simulink model "PIL_Block"  (R2017a)
settings: Solver=FixedStepAuto  StartTime=0.0  StopTime=50  FixedStep=0.01  RelTol=1e-3  EnableMultiTasking=on
libraries: pil_lib x1
settings Model: Creator=Administrator  LastModifiedBy=Administrator
settings OptimizationCC: PassReuseOutputArgsAs=Individual arguments  MaxStackSize=64
settings DebuggingCC: ParameterTunabilityLossMsg=error
settings HardwareCC: ProdBitPerPointer=32  ProdBitPerSizeT=32  ProdBitPerPtrDiffT=32  ProdLargestAtomicInteger=Long  ProdLargestAtomicFloat=Double  ProdWordSize=32  ProdHWDeviceType=ARM Compatible->ARM Cortex
settings SFSimCC: MATLABDynamicMemAlloc=off
settings RTWCC: SystemTargetFile=ert.tlc  HardwareBoard=ARM Cortex-M3 (QEMU)  TLCOptions=-aInlineSetEventsForThisBaseRateFcn=TLC_FALSE -aSuppressMultiTaskScheduler=TLC_FALSE -aRateBasedStepFcn=1  TemplateMakefile=ert_default_tmf  Description=Embedded Coder  GenerateReport=on  Toolchain=GNU Tools for ARM Embedded Processors  IncludeHyperlinkInReport=on  LaunchReport=on  CreateSILPILBlock=PIL  GenerateTraceInfo=on  GenerateTraceReport=on  GenerateTraceReportSl=on  GenerateTraceReportSf=on  GenerateTraceReportEml=on
settings CodeAppCC: ForceParamTrailComments=on  IgnoreCustomStorageClasses=off  OperatorAnnotations=on  SimulinkDataObjDesc=on  SFDataObjDesc=on  MATLABFcnDesc=on  InsertBlockDesc=on  MATLABSourceComments=on

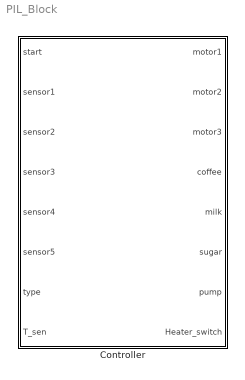
== system PIL_Block ==
  Controller : Subsystem  DialogController=pil_create_dialog  LoadFcn=|
      | try
      |    if ~strcmp(rtw.pil.getPILVersion, '6.12 (R2017a)_12')
      |       set_param(gcb, 'DialogController', '');
      |       set_param(gcb, 'DialogControllerArgs', '');
      |    end
      | catch e
      |       set_param(gcb, 'DialogController', '');
      |       set_param(gcb, 'DialogControllerArgs', '');
      | end
      mask help: PIL:pil:XILBlockMaskDesc
      mask Display: disp('PIL');

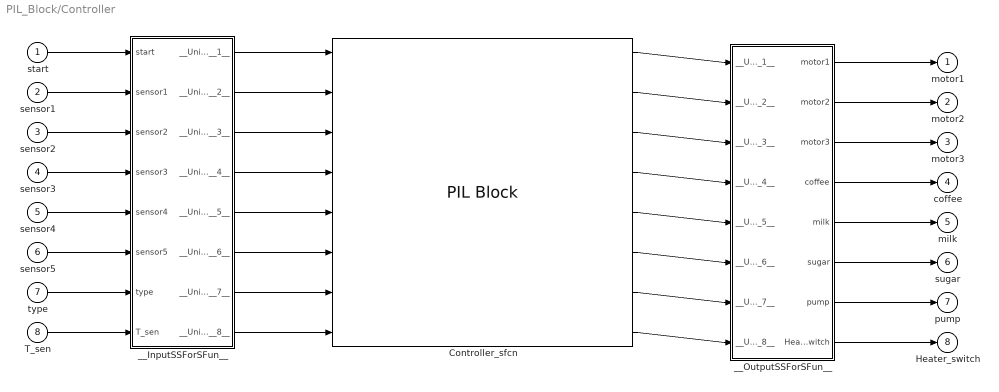
== system PIL_Block/Controller ==
  start : Inport
  sensor1 : Inport  Port=2
  sensor2 : Inport  Port=3
  sensor3 : Inport  Port=4
  sensor4 : Inport  Port=5
  sensor5 : Inport  Port=6
  type : Inport  Port=7
  T_sen : Inport  Port=8
  Controller_sfcn : pil_lib/PIL Block  SimulationMode=PIL  IsTopModelPIL=off  CodeDir=C:\Users\Administrator\Documents\MATLAB\Controller_ert_rtw  ConfigName=ARM Cortex-M3 (QEMU)  XrelIsTopModelCode=on
  __InputSSForSFun__ : Subsystem
  __OutputSSForSFun__ : Subsystem
  motor1 : Outport
  motor2 : Outport  Port=2
  motor3 : Outport  Port=3
  coffee : Outport  Port=4
  milk : Outport  Port=5
  sugar : Outport  Port=6
  pump : Outport  Port=7
  Heater_switch : Outport  Port=8
  wires:
  start/1 -> __InputSSForSFun__/1(start)
  sensor1/1 -> __InputSSForSFun__/2(sensor1)
  sensor2/1 -> __InputSSForSFun__/3(sensor2)
  sensor3/1 -> __InputSSForSFun__/4(sensor3)
  sensor4/1 -> __InputSSForSFun__/5(sensor4)
  sensor5/1 -> __InputSSForSFun__/6(sensor5)
  type/1 -> __InputSSForSFun__/7(type)
  T_sen/1 -> __InputSSForSFun__/8(T_sen)
  __InputSSForSFun__/1(__UniqueOutportName__1__) -> Controller_sfcn/1
  __InputSSForSFun__/2(__UniqueOutportName__2__) -> Controller_sfcn/2
  __InputSSForSFun__/3(__UniqueOutportName__3__) -> Controller_sfcn/3
  __InputSSForSFun__/4(__UniqueOutportName__4__) -> Controller_sfcn/4
  __InputSSForSFun__/5(__UniqueOutportName__5__) -> Controller_sfcn/5
  __InputSSForSFun__/6(__UniqueOutportName__6__) -> Controller_sfcn/6
  __InputSSForSFun__/7(__UniqueOutportName__7__) -> Controller_sfcn/7
  __InputSSForSFun__/8(__UniqueOutportName__8__) -> Controller_sfcn/8
  Controller_sfcn/1 -> __OutputSSForSFun__/1(__UniqueInportName__1__)
  Controller_sfcn/2 -> __OutputSSForSFun__/2(__UniqueInportName__2__)
  Controller_sfcn/3 -> __OutputSSForSFun__/3(__UniqueInportName__3__)
  Controller_sfcn/4 -> __OutputSSForSFun__/4(__UniqueInportName__4__)
  Controller_sfcn/5 -> __OutputSSForSFun__/5(__UniqueInportName__5__)
  Controller_sfcn/6 -> __OutputSSForSFun__/6(__UniqueInportName__6__)
  Controller_sfcn/7 -> __OutputSSForSFun__/7(__UniqueInportName__7__)
  Controller_sfcn/8 -> __OutputSSForSFun__/8(__UniqueInportName__8__)
  __OutputSSForSFun__/1(motor1) -> motor1/1
  __OutputSSForSFun__/2(motor2) -> motor2/1
  __OutputSSForSFun__/3(motor3) -> motor3/1
  __OutputSSForSFun__/4(coffee) -> coffee/1
  __OutputSSForSFun__/5(milk) -> milk/1
  __OutputSSForSFun__/6(sugar) -> sugar/1
  __OutputSSForSFun__/7(pump) -> pump/1
  __OutputSSForSFun__/8(Heater_switch) -> Heater_switch/1

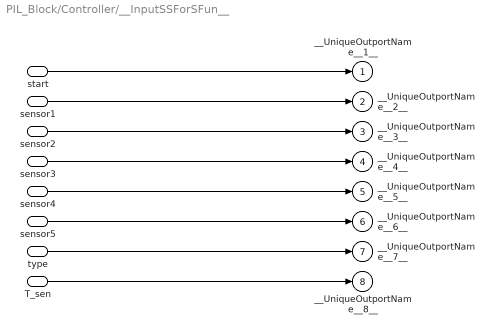
== system PIL_Block/Controller/__InputSSForSFun__ ==
  start : Inport
  sensor1 : Inport  Port=2
  sensor2 : Inport  Port=3
  sensor3 : Inport  Port=4
  sensor4 : Inport  Port=5
  sensor5 : Inport  Port=6
  type : Inport  Port=7
  T_sen : Inport  Port=8
  __UniqueOutportName__1__ : Outport
  __UniqueOutportName__2__ : Outport  Port=2
  __UniqueOutportName__3__ : Outport  Port=3
  __UniqueOutportName__4__ : Outport  Port=4
  __UniqueOutportName__5__ : Outport  Port=5
  __UniqueOutportName__6__ : Outport  Port=6
  __UniqueOutportName__7__ : Outport  Port=7
  __UniqueOutportName__8__ : Outport  Port=8
  wires:
  start/1 -> __UniqueOutportName__1__/1
  sensor1/1 -> __UniqueOutportName__2__/1
  sensor2/1 -> __UniqueOutportName__3__/1
  sensor3/1 -> __UniqueOutportName__4__/1
  sensor4/1 -> __UniqueOutportName__5__/1
  sensor5/1 -> __UniqueOutportName__6__/1
  type/1 -> __UniqueOutportName__7__/1
  T_sen/1 -> __UniqueOutportName__8__/1

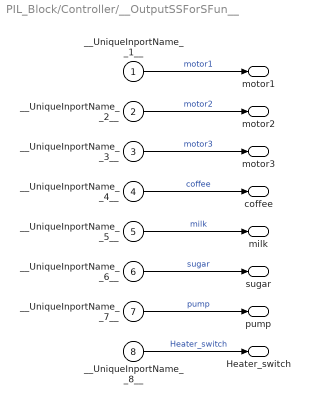
== system PIL_Block/Controller/__OutputSSForSFun__ ==
  __UniqueInportName__1__ : Inport
  __UniqueInportName__2__ : Inport  Port=2
  __UniqueInportName__3__ : Inport  Port=3
  __UniqueInportName__4__ : Inport  Port=4
  __UniqueInportName__5__ : Inport  Port=5
  __UniqueInportName__6__ : Inport  Port=6
  __UniqueInportName__7__ : Inport  Port=7
  __UniqueInportName__8__ : Inport  Port=8
  motor1 : Outport
  motor2 : Outport  Port=2
  motor3 : Outport  Port=3
  coffee : Outport  Port=4
  milk : Outport  Port=5
  sugar : Outport  Port=6
  pump : Outport  Port=7
  Heater_switch : Outport  Port=8
  wires:
  __UniqueInportName__1__/1 -> motor1/1  "motor1"
  __UniqueInportName__2__/1 -> motor2/1  "motor2"
  __UniqueInportName__3__/1 -> motor3/1  "motor3"
  __UniqueInportName__4__/1 -> coffee/1  "coffee"
  __UniqueInportName__5__/1 -> milk/1  "milk"
  __UniqueInportName__6__/1 -> sugar/1  "sugar"
  __UniqueInportName__7__/1 -> pump/1  "pump"
  __UniqueInportName__8__/1 -> Heater_switch/1  "Heater_switch"
